simulink model "Orbit_Sim_ECEF"  (R2017b)
settings: Solver=FixedStepAuto  StartTime=0.0  StopTime=stopTime  FixedStep=stepSize  RelTol=1e-3
values from neighbouring files (symbols this model uses):
  a = a_d    (= 6782.423)    [AA279D_hw4.m]    (also in AA279D_hw4_v2.m = 7500; SCHAUBprop.m = oe(1); TLE_Reader.m = (mu/n^2)^(1/3); keplerUniversal.m = 1./alpha(idx))
  e = 0    [AA279D_PSET3.m]    (also in AA279D_PSET4.m = 0.1; AA279D_hw4.m = 0.7; AA279D_hw4_v2.m = 0.1; SCHAUBprop.m = oe(2))
  inc = deg2rad(38.961)    [AA279D_hw4_v2.m]    (also in TLE_Reader.m = L3(1,3); test_space.mat = 51.6438)
  M0 = M    [AA279D_FINAL.m]    (also in AA279D_PSET1.m; AA279D_PSET2.m; AA279D_PSET2_a_change.m; AA279D_PSET3.m)
  n = n_D    [AA279D_hw4.m]    (also in AA279D_hw4_v2.m = sqrt(mu/a^3); AA279D_hw5_dv.m = sqrt(mu/at^3); OE2ECI.m = sqrt(mu/a^3); TLE_Reader.m = revs_per_day*2*pi/(24*3600))
  RAAN = 0    [AA279D_FINAL.m]    (also in AA279D_hw4_v2.m = deg2rad(358.1559); TLE_Reader.m = L3(1,4); test_space.mat = 331.1221)
  tol = 10^-5    (= 1e-05)    [AA279D_FINAL.m]    (also in AA279D_PSET1.m; AA279D_PSET2.m; AA279D_PSET2_a_change.m; AA279D_PSET3.m)
  w = 0    [AA279D_FINAL.m]    (also in AA279D_hw4.m = w_d; AA279D_hw4_v2.m = deg2rad(358.729); SCHAUBprop.m = oe(5); TLE_Reader.m = L3(1,6))
libraries: simulink_extras x4
settings Model: Creator=Patipan  LastModifiedBy=cwcovert

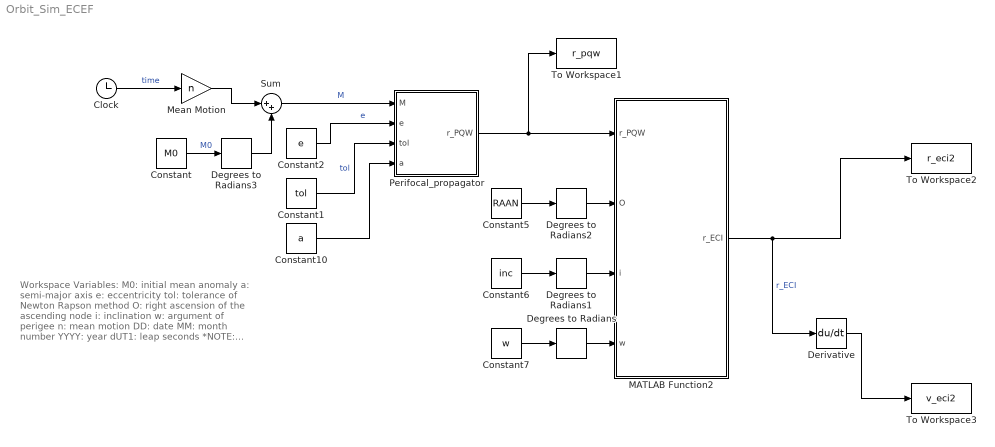
== system Orbit_Sim_ECEF ==
  note: Workspace Variables:
      | M0: initial mean anomaly
      | a: semi-major axis
      | e: eccentricity
      | tol: tolerance of Newton Rapson method
      | O: right ascension of the ascending node
      | i: inclination
      | w: argument of perigee
      | n: mean motion
      | DD: date
      | MM: month number
      | YYYY: year
      | dUT1: leap seconds
      |
      | *NOTE: angles are in radians
  Clock : Clock
  Constant : Constant  Value=M0
  Constant1 : Constant  Value=tol
  Constant10 : Constant  Value=a
  Constant2 : Constant  Value=e
  Constant5 : Constant  Value=RAAN
  Constant6 : Constant  Value=inc
  Constant7 : Constant  Value=w
  Degrees to Radians{,1..3} (4 alike) : simulink_extras/Transformations/Degrees to Radians
  Derivative : Derivative
  MATLAB Function2 : MATLAB Function  TreatAsAtomicUnit=on
  Mean Motion : Gain  Gain=n
  Perifocal_propagator : Subsystem
  Sum : Sum  Inputs=|++
  To Workspace1 : ToWorkspace  VariableName=r_pqw  SampleTime=-1
  To Workspace2 : ToWorkspace  VariableName=r_eci2  SampleTime=-1
  To Workspace3 : ToWorkspace  VariableName=v_eci2  SampleTime=-1
  wires:
  Clock/1 -> Mean Motion/1  "time"
  MATLAB Function2/1(r_ECI) -> Derivative/1, To Workspace2/1  "r_ECI"
  Sum/1 -> Perifocal_propagator/1(M)  "M"
  Constant2/1 -> Perifocal_propagator/2(e)  "e"
  Constant1/1 -> Perifocal_propagator/3(tol)  "tol"
  Perifocal_propagator/1(r_PQW) -> To Workspace1/1, MATLAB Function2/1(r_PQW)
  Constant10/1 -> Perifocal_propagator/4(a)
  Constant5/1 -> Degrees to Radians2/1
  Degrees to Radians2/1 -> MATLAB Function2/2(O)
  Degrees to Radians1/1 -> MATLAB Function2/3(i)
  Constant6/1 -> Degrees to Radians1/1
  Constant7/1 -> Degrees to Radians/1
  Degrees to Radians/1 -> MATLAB Function2/4(w)
  Constant/1 -> Degrees to Radians3/1  "M0"
  Degrees to Radians3/1 -> Sum/2
  Derivative/1 -> To Workspace3/1
  Mean Motion/1 -> Sum/1

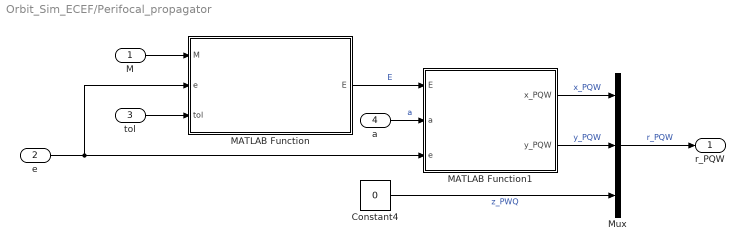
== system Orbit_Sim_ECEF/Perifocal_propagator ==
  M : Inport
  e : Inport  Port=2
  tol : Inport  Port=3
  a : Inport  Port=4
  Constant4 : Constant  Value=0
  MATLAB Function : MATLAB Function  TreatAsAtomicUnit=on
  MATLAB Function1 : MATLAB Function  TreatAsAtomicUnit=on
  Mux : Mux  Inputs=3
  r_PQW : Outport
  wires:
  tol/1 -> MATLAB Function/3(tol)
  MATLAB Function/1(E) -> MATLAB Function1/1(E)  "E"
  M/1 -> MATLAB Function/1(M)
  e/1 -> MATLAB Function1/3(e), MATLAB Function/2(e)
  a/1 -> MATLAB Function1/2(a)  "a"
  MATLAB Function1/1(x_PQW) -> Mux/1  "x_PQW"
  MATLAB Function1/2(y_PQW) -> Mux/2  "y_PQW"
  Constant4/1 -> Mux/3  "z_PWQ"
  Mux/1 -> r_PQW/1  "r_PQW"

== matlab function Orbit_Sim_ECEF/Perifocal_propagator/MATLAB Function1 ==
  data: x_PQW output; E input; y_PQW output; a input; e input
function [x_PQW, y_PQW] = E2Pos(E, a, e)

% Compute position in perifocal coordinates
%
% Inputs
% ------
% E         Eccentric anomaly
% a         semi-major axis
%
% Outputs
% -------
% x         x position on orbital plane
% y         y position on orbital plane

% semi-latus rectum
p = a*(1 - e^2);

% Compute true anomaly from eccentric anomaly
cos_nu = (cos(E) - e) / (1 - e*cos(E));
sin_nu = (sin(E)*sqrt(1 - e^2)) / (1 - e*cos(E));
nu = atan2(sin_nu, cos_nu);

% Compute radial position
r = p / (1 + e*cos(nu));

% convert to cartesian
x_PQW = r*cos(nu);
y_PQW = r*sin(nu);

== matlab function Orbit_Sim_ECEF/Perifocal_propagator/MATLAB Function ==
  data: M input; e input; E output; tol input
function E = MeanAnom2EccAnom(M, e, tol) 

% Compute eccentric anomaly from mean anomaly
%
% Inputs
% ------
% M         mean anomaly [rad]
% e         eccentricity
% tol       tolerance
%
% Outputs
% -------
% E         Eccentric anomaly [rad]
% v         velocity vector

% Check edge cases
if( M == pi || M == 0)
    E = M;
    return
end

% initial guess
if( M > pi )
    E = M - e/2;
else
    E = M + e/2;
end

err = 1;
count = 0;
while err > tol
    % Compute correction value
    delta = -(E - e*sin(E) - M)/(1 - e*cos(E));

    % Error
    err = abs(delta);
  
    E = E + delta;
    
    % Limit # of iterations
    count = count + 1;
    if count > 1e6
        return
    end
end

== matlab function Orbit_Sim_ECEF/MATLAB Function2 ==
  data: r_PQW input; r_ECI output; O input; i input; w input
function r_ECI = PQW2ECI(r_PQW, O, i, w)

% Transform vector in perifocal to ECI
%
% Inputs
% ------
% r_PQW     position in perifocal coordinates
% i         inclination [rad]
% O       	right ascension of ascending node [rad]
% w         argument of pariapsis [rad]
%
% Outputs
% -------
% r_ECI     position in ECI coordinates

% Compute rotation matrix from PQW to ECI (3-1-3 Euler rots)
Rz_O = [cos(-O)     sin(-O)     0;
        -sin(-O)    cos(-O)     0;
        0           0           1;];
Rx_i = [1   0           0;
        0   cos(-i)     sin(-i);
        0   -sin(-i)    cos(-i);];
Rz_w = [cos(-w)     sin(-w)     0;
        -sin(-w)    cos(-w)     0;
        0           0           1;];
R_PWQ2ECI = Rz_O * Rx_i * Rz_w;

r_ECI = R_PWQ2ECI * r_PQW;
